simulink model "gm_sampleModel1517_2_sub"  (R2023a)
settings: Solver=VariableStepAuto  StartTime=0.0  StopTime=10.0  RelTol=1e-3
libraries: simulink x1
settings Model: Creator=user1  LastModifiedBy=user1
settings OptimizationCC: BlockReduction=off  ConditionallyExecuteInputs=off
settings DebuggingCC: InheritedTsInSrcMsg=none

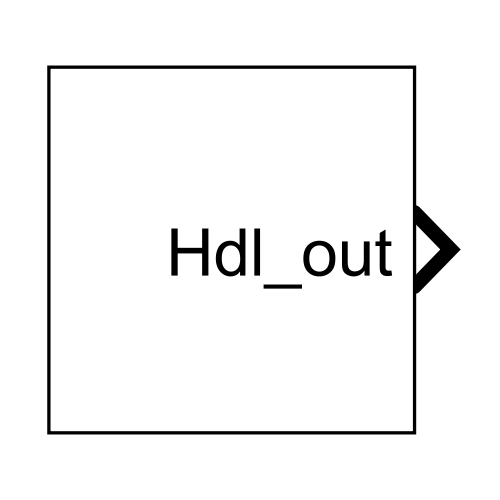
[thumbnail: Simulink's stored preview of the top-level diagram]
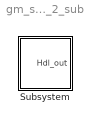
== system gm_sampleModel1517_2_sub ==
  Subsystem : Subsystem

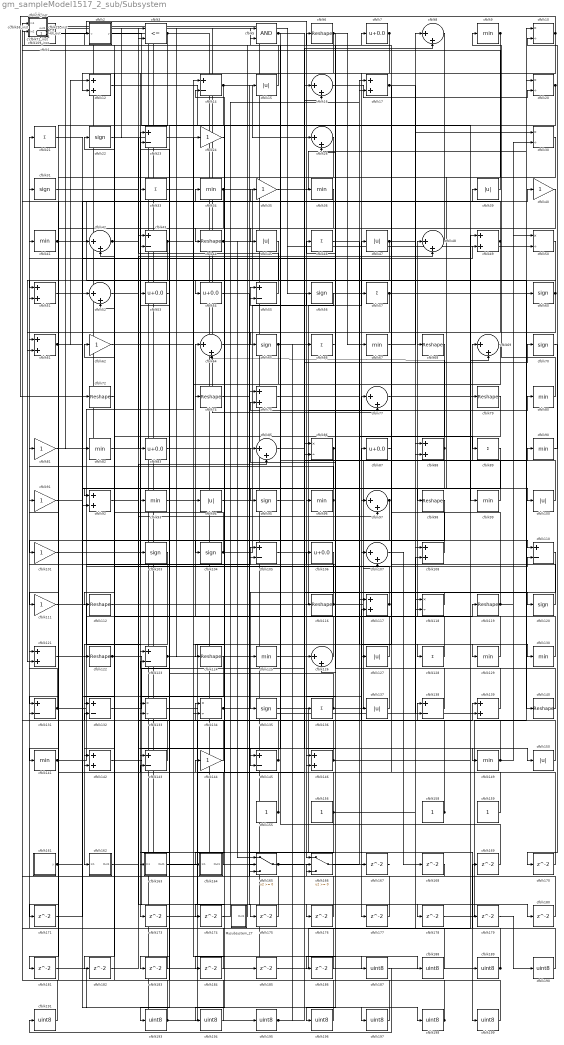
== system gm_sampleModel1517_2_sub/Subsystem ==
  Mysubsystem_27 : Subsystem
  cfblk1 : simulink/Logic and Bit Operations/Extract Bits  bitsToExtract=Upper half  numBits=8  bitIdxRange=[0 7]  outScalingMode=Preserve fixed-point scaling
      settings: LibrarySourceBlock=|
      | hdlsllib/Logic and Bit
      | Operations/Extract Bits
  cfblk{10,20,30,50,86,118,133..134} (8 alike) : Product  Inputs=*/  OutDataTypeStr=uint8  RndMeth=Zero  SaturateOnIntegerOverflow=on
  cfblk{15,39,45,47,94,100,127,137,150} (9 alike) : Abs  OutDataTypeStr=uint8  SaturateOnIntegerOverflow=off
  cfblk{24,35,40,62,81,91,101,111,144} (9 alike) : Gain  OutDataTypeStr=uint8
  cfblk102_inst : Subsystem
  cfblk{22,31,56,60,65,70,95,103..104,120,135} (11 alike) : Signum
  cfblk{14,23,43,55,105,110,123,131..132,138,143,145} (12 alike) : Sum  Inputs=+-  OutDataTypeStr=uint8
  cfblk{7,53..54,83,87,106} (6 alike) : Bias  Bias=0.0  SaturateOnIntegerOverflow=off
  cfblk{8,16,26,42,48,52,64,69,77,85,97,107,126} (13 alike) : Sum  Inputs=|++  OutDataTypeStr=uint8
  cfblk{12,17,49,51,61,75,88,92,108,117,121,139,142,146} (14 alike) : Sum  OutDataTypeStr=uint8
  cfblk109_inst : Subsystem
  cfblk{6,44,68,72,74,79,98,112,116,119,122,124,140} (13 alike) : Reshape
  cfblk{9,34,36,41,67,80,82,90,93,96,99,125,129..130,141,149} (16 alike) : MinMax  OutDataTypeStr=uint8
  cfblk{21,33,46,57,66,89,128,136} (8 alike) : Sum  Inputs=+  OutDataTypeStr=uint8
  cfblk147_inst : Subsystem
  cfblk{155..156,158..159} (4 alike) : Constant  OutDataTypeStr=uint8  SampleTime=-1
  cfblk161 : Subsystem  mask(Counter Free-Running){NumBits=double(16), tsamp=double(-1)}
      mask prompts: NumBits "Simulink:masks:NumberOfBits_MP"; tsamp "Simulink:masks:SampleTime_MP"
      mask help: Simulink:masks:CounterFreeRunning_MD
  cfblk162 : Subsystem
  cfblk163 : Subsystem
  cfblk164 : Subsystem
  cfblk165 : Switch  OutDataTypeStr=uint8  SaturateOnIntegerOverflow=off  InputSameDT=off
  cfblk166 : Switch  OutDataTypeStr=uint8  SaturateOnIntegerOverflow=off  InputSameDT=off
  cfblk{167..171,173..186} (19 alike) : Delay  SampleTime=1
  cfblk{187..191,193..199} (12 alike) : DataTypeConversion  OutDataTypeStr=uint8  SaturateOnIntegerOverflow=off  RndMeth=Floor
  cfblk19_inst : Subsystem
  cfblk2 : Subsystem  mask(Compare To Zero){relop=<=, OutDataTypeStr=uint8, ZeroCross=on}
      mask prompts: relop "Simulink:masks:Operator_MP"; OutDataTypeStr "Simulink:masks:OutputDataType_MP"; ZeroCross "Simulink:masks:EnableZerocrossingDetection_MP"
      mask help: Simulink:masks:CompareToZero_MD
      mask init:
      | OutDataTypeStr = 'uint8';
      | ZeroCross = 'on';
      | blkName = 'sampleModel1517_2_sub/Subsystem/cfblk2';
      | relop = '<=';
      | setValue = 'fixdt(0, 8)';
      mask TypeOptions relop: == | ~= | < | <= | >= | >
      mask TypeOptions OutDataTypeStr: Simulink:masks:uint8 | Simulink:masks:boolean
      mask Callback ZeroCross: sl('zeroCrossEnable', gcbh);
      mask Display: disp([relop,' 0'])
  cfblk29_inst : Subsystem
  cfblk3 : RelationalOperator  Operator=<=  OutDataTypeStr=boolean  InputSameDT=off
  cfblk4 : Constant  Value=0  OutDataTypeStr=uint8  SampleTime=1
  cfblk5 : Logic  AllPortsSameDT=off  OutDataTypeStr=boolean
  cfblk58_inst : Subsystem
  cfblk71_inst : Subsystem
  Hdl_out : Outport  OutDataTypeStr=uint8  SampleTime=1
  wires:
  Mysubsystem_27/1(Out1) -> cfblk71_inst/2(in2)
  cfblk1/1 -> cfblk166/1
  cfblk10/1 -> cfblk72/1, cfblk177/1, cfblk173/1
  cfblk100/1 -> cfblk69/1
  cfblk101/1 -> cfblk23/1
  cfblk102_inst/1(out1) -> cfblk24/1, cfblk185/1
  cfblk103/1 -> cfblk162/1(In1)
  cfblk104/1 -> cfblk56/1, cfblk22/1
  cfblk105/1 -> cfblk80/1
  cfblk106/1 -> cfblk135/1
  cfblk107/1 -> cfblk168/1
  cfblk108/1 -> cfblk87/1
  cfblk109_inst/1(out1) -> cfblk126/1
  cfblk110/1 -> cfblk126/2
  cfblk111/1 -> cfblk123/1
  cfblk112/1 -> cfblk47/1
  cfblk116/1 -> cfblk48/1, cfblk21/1
  cfblk117/1 -> cfblk64/1, cfblk42/2
  cfblk118/1 -> cfblk116/1
  cfblk119/1 -> cfblk75/2, cfblk109_inst/2(in2), cfblk50/1
  cfblk12/1 -> cfblk79/1
  cfblk120/1 -> cfblk33/1
  cfblk121/1 -> cfblk119/1
  cfblk122/1 -> cfblk97/2, cfblk176/1
  cfblk123/1 -> cfblk178/1, cfblk128/1
  cfblk124/1 -> cfblk183/1
  cfblk125/1 -> cfblk8/2
  cfblk126/1 -> cfblk23/2
  cfblk127/1 -> cfblk106/1
  cfblk128/1 -> cfblk68/1
  cfblk129/1 -> cfblk74/1
  cfblk130/1 -> cfblk2/1(u)
  cfblk131/1 -> cfblk51/2, cfblk110/2
  cfblk132/1 -> cfblk90/1
  cfblk133/1 -> cfblk175/1
  cfblk134/1 -> cfblk165/2, cfblk34/1
  cfblk135/1 -> cfblk199/1
  cfblk136/1 -> cfblk107/2, cfblk103/1
  cfblk137/1 -> cfblk105/1
  cfblk138/1 -> cfblk41/1
  cfblk139/1 -> cfblk85/1
  cfblk14/1 -> cfblk26/1, cfblk163/1(In1)
  cfblk140/1 -> cfblk6/1
  cfblk141/1 -> cfblk14/1, cfblk105/2
  cfblk142/1 -> cfblk167/1
  cfblk143/1 -> cfblk147_inst/1(in1)
  cfblk144/1 -> cfblk58_inst/2(in2)
  cfblk145/1 -> cfblk143/1, cfblk134/1
  cfblk146/1 -> cfblk49/1, cfblk62/1
  cfblk147_inst/1(out1) -> cfblk83/1
  cfblk149/1 -> cfblk117/2, cfblk30/2
  cfblk15/1 -> cfblk5/1
  cfblk150/1 -> cfblk138/1
  cfblk155/1 -> cfblk31/1, cfblk143/2
  cfblk156/1 -> cfblk55/1, cfblk165/3, cfblk108/2
  cfblk158/1 -> cfblk61/1, cfblk117/1
  cfblk159/1 -> cfblk77/1
  cfblk16/1 -> cfblk20/2
  cfblk161/1(y) -> cfblk49/2, cfblk40/1
  cfblk162/1(Out1) -> cfblk139/1
  cfblk163/1(Out1) -> cfblk15/1
  cfblk164/1(Out1) -> cfblk144/1
  cfblk165/1 -> cfblk16/1, Hdl_out/1
  cfblk166/1 -> cfblk17/2
  cfblk167/1 -> cfblk1/1
  cfblk168/1 -> cfblk166/2
  cfblk169/1 -> cfblk5/2
  cfblk17/1 -> cfblk118/2, cfblk57/1
  cfblk170/1 -> cfblk14/2
  cfblk171/1 -> cfblk52/1
  cfblk173/1 -> cfblk16/2
  cfblk174/1 -> cfblk17/1
  cfblk175/1 -> cfblk75/1
  cfblk176/1 -> cfblk123/2
  cfblk177/1 -> cfblk166/3
  cfblk178/1 -> cfblk20/1
  cfblk179/1 -> cfblk190/1
  cfblk180/1 -> cfblk58_inst/1(in1)
  cfblk181/1 -> cfblk197/1
  cfblk182/1 -> cfblk85/2
  cfblk183/1 -> cfblk121/1
  cfblk184/1 -> cfblk131/2
  cfblk185/1 -> cfblk69/2
  cfblk186/1 -> cfblk43/2
  cfblk187/1 -> cfblk191/1
  cfblk188/1 -> cfblk93/1
  cfblk189/1 -> cfblk169/1, cfblk118/1
  cfblk19_inst/1(out1) -> cfblk195/1
  cfblk190/1 -> cfblk29_inst/1(in1)
  cfblk191/1 -> cfblk29_inst/2(in2)
  cfblk193/1 -> cfblk71_inst/1(in1), cfblk86/2
  cfblk194/1 -> cfblk53/1
  cfblk195/1 -> cfblk86/1, cfblk66/1
  cfblk196/1 -> cfblk19_inst/1(in1)
  cfblk197/1 -> cfblk19_inst/2(in2)
  cfblk198/1 -> cfblk132/2, cfblk109_inst/1(in1)
  cfblk199/1 -> cfblk91/1
  cfblk2/1(y) -> cfblk88/1
  cfblk20/1 -> cfblk196/1, cfblk184/1
  cfblk21/1 -> cfblk110/1
  cfblk22/1 -> cfblk43/1
  cfblk23/1 -> cfblk94/1
  cfblk24/1 -> cfblk44/1
  cfblk26/1 -> cfblk101/1
  cfblk29_inst/1(out1) -> cfblk189/1
  cfblk3/1 -> cfblk92/1, cfblk181/1
  cfblk30/1 -> cfblk98/1
  cfblk31/1 -> cfblk146/2
  cfblk33/1 -> cfblk188/1
  cfblk34/1 -> cfblk108/1, cfblk171/1
  cfblk35/1 -> cfblk10/1
  cfblk36/1 -> cfblk194/1
  cfblk39/1 -> cfblk102_inst/2(in2)
  cfblk4/1 -> cfblk139/2
  cfblk40/1 -> cfblk127/1
  cfblk41/1 -> cfblk140/1, cfblk35/1
  cfblk42/1 -> cfblk3/2, cfblk182/1
  cfblk43/1 -> cfblk112/1, cfblk130/1
  cfblk44/1 -> cfblk88/2, cfblk165/1
  cfblk45/1 -> cfblk61/2
  cfblk46/1 -> cfblk129/1
  cfblk47/1 -> cfblk138/2, cfblk131/1
  cfblk48/1 -> cfblk45/1
  cfblk49/1 -> cfblk102_inst/1(in1), cfblk133/2
  cfblk5/1 -> cfblk145/2, cfblk120/1
  cfblk50/1 -> cfblk107/1
  cfblk51/1 -> cfblk96/1
  cfblk52/1 -> cfblk54/1
  cfblk53/1 -> cfblk193/1
  cfblk54/1 -> cfblk145/1
  cfblk55/1 -> cfblk3/1
  cfblk56/1 -> cfblk55/2
  cfblk57/1 -> cfblk8/1, cfblk121/2
  cfblk58_inst/1(out1) -> cfblk60/1, cfblk82/1
  cfblk6/1 -> cfblk142/2, cfblk186/1, cfblk67/1
  cfblk60/1 -> cfblk65/1, cfblk51/1, cfblk136/1
  cfblk61/1 -> cfblk137/1, cfblk12/1
  cfblk62/1 -> cfblk97/1
  cfblk64/1 -> cfblk179/1
  cfblk65/1 -> cfblk150/1, cfblk134/2
  cfblk66/1 -> cfblk46/1
  cfblk67/1 -> cfblk30/1
  cfblk68/1 -> cfblk132/1
  cfblk69/1 -> cfblk104/1
  cfblk7/1 -> cfblk12/2, cfblk36/1
  cfblk70/1 -> cfblk170/1
  cfblk71_inst/1(out1) -> cfblk77/2, cfblk50/2
  cfblk72/1 -> cfblk122/1
  cfblk74/1 -> cfblk149/1
  cfblk75/1 -> cfblk89/1
  cfblk77/1 -> cfblk99/1
  cfblk79/1 -> cfblk146/1
  cfblk8/1 -> cfblk142/1
  cfblk80/1 -> cfblk9/1
  cfblk81/1 -> cfblk42/1
  cfblk82/1 -> cfblk48/2
  cfblk83/1 -> cfblk39/1
  cfblk85/1 -> cfblk100/1
  cfblk86/1 -> cfblk26/2, cfblk124/1
  cfblk87/1 -> cfblk7/1
  cfblk88/1 -> cfblk92/2, cfblk64/2
  cfblk89/1 -> cfblk164/1(In1)
  cfblk9/1 -> cfblk95/1, cfblk52/2
  cfblk90/1 -> cfblk10/2
  cfblk91/1 -> cfblk198/1
  cfblk92/1 -> cfblk180/1
  cfblk93/1 -> cfblk187/1
  cfblk94/1 -> cfblk125/1
  cfblk95/1 -> cfblk70/1
  cfblk96/1 -> cfblk81/1, cfblk141/1
  cfblk97/1 -> cfblk174/1, cfblk133/1
  cfblk98/1 -> cfblk111/1
  cfblk99/1 -> cfblk147_inst/2(in2)

== system gm_sampleModel1517_2_sub/Subsystem/Mysubsystem_27 ==
  cfblk157 : Subsystem  mask(Counter Free-Running){NumBits=double(16), tsamp=double(-1)}
      mask prompts: NumBits "Simulink:masks:NumberOfBits_MP"; tsamp "Simulink:masks:SampleTime_MP"
      mask help: Simulink:masks:CounterFreeRunning_MD
  cfblk192 : DataTypeConversion  OutDataTypeStr=uint8  SaturateOnIntegerOverflow=off  RndMeth=Floor
  Out1 : Outport  SampleTime=1
  wires:
  cfblk157/1(y) -> cfblk192/1
  cfblk192/1 -> Out1/1

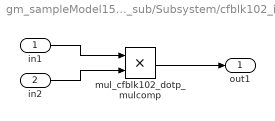
== system gm_sampleModel1517_2_sub/Subsystem/cfblk102_inst ==
  in1 : Inport  OutDataTypeStr=uint8  SampleTime=1
  in2 : Inport  Port=2  OutDataTypeStr=uint8  SampleTime=1
  mul_cfblk102_dotp_mulcomp : Product  Inputs=**  OutDataTypeStr=uint8  SampleTime=1
  out1 : Outport  OutDataTypeStr=uint8  SampleTime=1
  wires:
  in1/1 -> mul_cfblk102_dotp_mulcomp/1
  in2/1 -> mul_cfblk102_dotp_mulcomp/2
  mul_cfblk102_dotp_mulcomp/1 -> out1/1

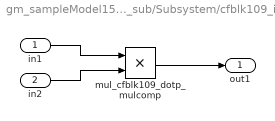
== system gm_sampleModel1517_2_sub/Subsystem/cfblk109_inst ==
  in1 : Inport  OutDataTypeStr=uint8  SampleTime=1
  in2 : Inport  Port=2  OutDataTypeStr=uint8  SampleTime=1
  mul_cfblk109_dotp_mulcomp : Product  Inputs=**  OutDataTypeStr=uint8  SampleTime=1
  out1 : Outport  OutDataTypeStr=uint8  SampleTime=1
  wires:
  in1/1 -> mul_cfblk109_dotp_mulcomp/1
  in2/1 -> mul_cfblk109_dotp_mulcomp/2
  mul_cfblk109_dotp_mulcomp/1 -> out1/1

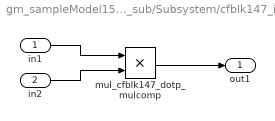
== system gm_sampleModel1517_2_sub/Subsystem/cfblk147_inst ==
  in1 : Inport  OutDataTypeStr=uint8  SampleTime=1
  in2 : Inport  Port=2  OutDataTypeStr=uint8  SampleTime=1
  mul_cfblk147_dotp_mulcomp : Product  Inputs=**  OutDataTypeStr=uint8  SampleTime=1
  out1 : Outport  OutDataTypeStr=uint8  SampleTime=1
  wires:
  in1/1 -> mul_cfblk147_dotp_mulcomp/1
  in2/1 -> mul_cfblk147_dotp_mulcomp/2
  mul_cfblk147_dotp_mulcomp/1 -> out1/1

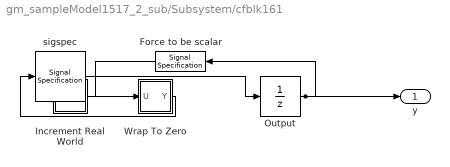
== system gm_sampleModel1517_2_sub/Subsystem/cfblk161 ==
  Force to be scalar : SignalSpecification  DisableCoverage=on  Dimensions=1
  Increment Real World : Subsystem  mask(Real World Value Increment){}
      mask help: Simulink:masks:RealWorldValueIncrement_MD
      mask Display: disp('V++')
  Output : UnitDelay  InitialCondition=0.0  SampleTime=tsamp  HasFrameUpgradeWarning=on
  Wrap To Zero : Subsystem  mask(Wrap To Zero){Threshold=double(65535)}
      mask prompts: Threshold "Simulink:masks:Threshold_MP"
      mask help: Simulink:masks:WrapToZero_MD
  sigspec : SignalSpecification  OutDataTypeStr=uint16  Dimensions=1
  y : Outport  SampleTime=1
  wires:
  Force to be scalar/1 -> Increment Real World/1(u)
  Increment Real World/1(y) -> Wrap To Zero/1(U)
  Output/1 -> Force to be scalar/1, y/1
  Wrap To Zero/1(Y) -> sigspec/1
  sigspec/1 -> Output/1

== system gm_sampleModel1517_2_sub/Subsystem/cfblk162 ==
  In1 : Inport  OutDataTypeStr=uint8  PortDimensions=1  SampleTime=1
  Out1 : Outport  SampleTime=1
  wires:
  In1/1 -> Out1/1

== system gm_sampleModel1517_2_sub/Subsystem/cfblk163 ==
  In1 : Inport  OutDataTypeStr=uint8  PortDimensions=1  SampleTime=1
  Out1 : Outport  SampleTime=1
  wires:
  In1/1 -> Out1/1

== system gm_sampleModel1517_2_sub/Subsystem/cfblk164 ==
  In1 : Inport  OutDataTypeStr=uint8  PortDimensions=1  SampleTime=1
  Out1 : Outport  SampleTime=1
  wires:
  In1/1 -> Out1/1

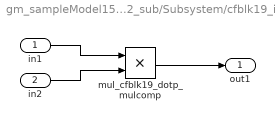
== system gm_sampleModel1517_2_sub/Subsystem/cfblk19_inst ==
  in1 : Inport  OutDataTypeStr=uint8  SampleTime=1
  in2 : Inport  Port=2  OutDataTypeStr=uint8  SampleTime=1
  mul_cfblk19_dotp_mulcomp : Product  Inputs=**  OutDataTypeStr=uint8  SampleTime=1
  out1 : Outport  OutDataTypeStr=uint8  SampleTime=1
  wires:
  in1/1 -> mul_cfblk19_dotp_mulcomp/1
  in2/1 -> mul_cfblk19_dotp_mulcomp/2
  mul_cfblk19_dotp_mulcomp/1 -> out1/1

== system gm_sampleModel1517_2_sub/Subsystem/cfblk2 ==
  u : Inport  OutDataTypeStr=uint8  SampleTime=1
  Compare : RelationalOperator  Operator=<=  OutDataTypeStr=fixdt(0, 8)
  Constant : Constant  DisableCoverage=on  Value=0  OutDataTypeStr=Inherit: Inherit via back propagation  SampleTime=-1  PreserveConstantTs=on
  y : Outport  SampleTime=1
  wires:
  u/1 -> Compare/1
  Compare/1 -> y/1
  Constant/1 -> Compare/2

== system gm_sampleModel1517_2_sub/Subsystem/cfblk29_inst ==
  in1 : Inport  OutDataTypeStr=uint8  SampleTime=1
  in2 : Inport  Port=2  OutDataTypeStr=uint8  SampleTime=1
  mul_cfblk29_dotp_mulcomp : Product  Inputs=**  OutDataTypeStr=uint8  SampleTime=1
  out1 : Outport  OutDataTypeStr=uint8  SampleTime=1
  wires:
  in1/1 -> mul_cfblk29_dotp_mulcomp/1
  in2/1 -> mul_cfblk29_dotp_mulcomp/2
  mul_cfblk29_dotp_mulcomp/1 -> out1/1

== system gm_sampleModel1517_2_sub/Subsystem/cfblk58_inst ==
  in1 : Inport  OutDataTypeStr=uint8  SampleTime=1
  in2 : Inport  Port=2  OutDataTypeStr=uint8  SampleTime=1
  mul_cfblk58_dotp_mulcomp : Product  Inputs=**  OutDataTypeStr=uint8  SampleTime=1
  out1 : Outport  OutDataTypeStr=uint8  SampleTime=1
  wires:
  in1/1 -> mul_cfblk58_dotp_mulcomp/1
  in2/1 -> mul_cfblk58_dotp_mulcomp/2
  mul_cfblk58_dotp_mulcomp/1 -> out1/1

== system gm_sampleModel1517_2_sub/Subsystem/cfblk71_inst ==
  in1 : Inport  OutDataTypeStr=uint8  SampleTime=1
  in2 : Inport  Port=2  OutDataTypeStr=uint8  SampleTime=1
  mul_cfblk71_dotp_mulcomp : Product  Inputs=**  OutDataTypeStr=uint8  SampleTime=1
  out1 : Outport  OutDataTypeStr=uint8  SampleTime=1
  wires:
  in1/1 -> mul_cfblk71_dotp_mulcomp/1
  in2/1 -> mul_cfblk71_dotp_mulcomp/2
  mul_cfblk71_dotp_mulcomp/1 -> out1/1

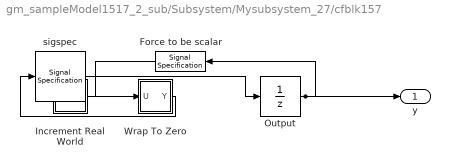
== system gm_sampleModel1517_2_sub/Subsystem/Mysubsystem_27/cfblk157 ==
  Force to be scalar : SignalSpecification  DisableCoverage=on  Dimensions=1
  Increment Real World : Subsystem  mask(Real World Value Increment){}
      mask help: Simulink:masks:RealWorldValueIncrement_MD
      mask Display: disp('V++')
  Output : UnitDelay  InitialCondition=0.0  SampleTime=tsamp  HasFrameUpgradeWarning=on
  Wrap To Zero : Subsystem  mask(Wrap To Zero){Threshold=double(65535)}
      mask prompts: Threshold "Simulink:masks:Threshold_MP"
      mask help: Simulink:masks:WrapToZero_MD
  sigspec : SignalSpecification  OutDataTypeStr=uint16  Dimensions=1
  y : Outport  SampleTime=1
  wires:
  Force to be scalar/1 -> Increment Real World/1(u)
  Increment Real World/1(y) -> Wrap To Zero/1(U)
  Output/1 -> Force to be scalar/1, y/1
  Wrap To Zero/1(Y) -> sigspec/1
  sigspec/1 -> Output/1

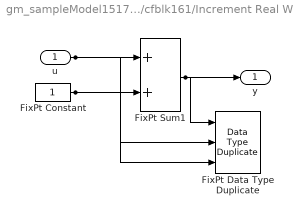
== system gm_sampleModel1517_2_sub/Subsystem/cfblk161/Increment Real World ==
  u : Inport  OutDataTypeStr=uint16  SampleTime=1
  FixPt Constant : Constant  DisableCoverage=on  OutDataTypeStr=Inherit: Inherit via back propagation  SampleTime=-1
  FixPt Data Type Duplicate : DataTypeDuplicate  DisableCoverage=on  NumInputPorts=3
  FixPt Sum1 : Sum  InputSameDT=on  OutDataTypeStr=Inherit: Inherit via back propagation  LockScale=on
  y : Outport  SampleTime=1
  wires:
  u/1 -> FixPt Sum1/1, FixPt Data Type Duplicate/2
  FixPt Constant/1 -> FixPt Sum1/2, FixPt Data Type Duplicate/3
  FixPt Sum1/1 -> FixPt Data Type Duplicate/1, y/1

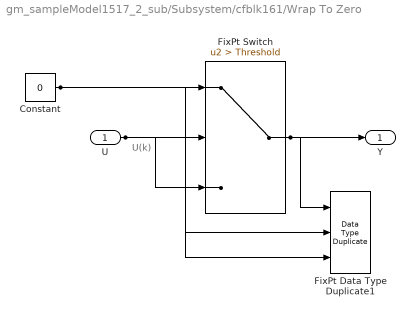
== system gm_sampleModel1517_2_sub/Subsystem/cfblk161/Wrap To Zero ==
  note: U(k)
  U : Inport  OutDataTypeStr=uint16  SampleTime=1
  Constant : Constant  DisableCoverage=on  Value=0  OutDataTypeStr=Inherit: Inherit via back propagation  SampleTime=-1
  FixPt Data Type Duplicate1 : DataTypeDuplicate  DisableCoverage=on  NumInputPorts=3
  FixPt Switch : Switch  Criteria=u2 > Threshold  Threshold=Threshold  OutDataTypeStr=Inherit: Inherit via back propagation  ZeroCross=off  SaturateOnIntegerOverflow=off  InputSameDT=off
  Y : Outport  SampleTime=1
  wires:
  U/1 -> FixPt Switch/3, FixPt Switch/2, FixPt Data Type Duplicate1/2
  Constant/1 -> FixPt Switch/1, FixPt Data Type Duplicate1/3
  FixPt Switch/1 -> FixPt Data Type Duplicate1/1, Y/1

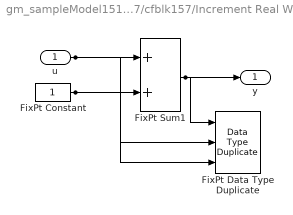
== system gm_sampleModel1517_2_sub/Subsystem/Mysubsystem_27/cfblk157/Increment Real World ==
  u : Inport  OutDataTypeStr=uint16  SampleTime=1
  FixPt Constant : Constant  DisableCoverage=on  OutDataTypeStr=Inherit: Inherit via back propagation  SampleTime=-1
  FixPt Data Type Duplicate : DataTypeDuplicate  DisableCoverage=on  NumInputPorts=3
  FixPt Sum1 : Sum  InputSameDT=on  OutDataTypeStr=Inherit: Inherit via back propagation  LockScale=on
  y : Outport  SampleTime=1
  wires:
  u/1 -> FixPt Sum1/1, FixPt Data Type Duplicate/2
  FixPt Constant/1 -> FixPt Sum1/2, FixPt Data Type Duplicate/3
  FixPt Sum1/1 -> FixPt Data Type Duplicate/1, y/1

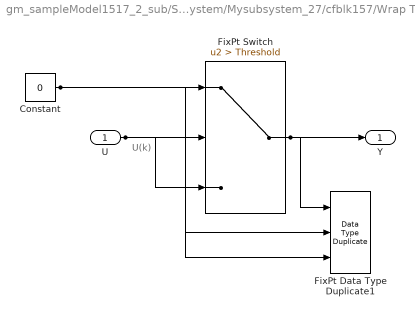
== system gm_sampleModel1517_2_sub/Subsystem/Mysubsystem_27/cfblk157/Wrap To Zero ==
  note: U(k)
  U : Inport  OutDataTypeStr=uint16  SampleTime=1
  Constant : Constant  DisableCoverage=on  Value=0  OutDataTypeStr=Inherit: Inherit via back propagation  SampleTime=-1
  FixPt Data Type Duplicate1 : DataTypeDuplicate  DisableCoverage=on  NumInputPorts=3
  FixPt Switch : Switch  Criteria=u2 > Threshold  Threshold=Threshold  OutDataTypeStr=Inherit: Inherit via back propagation  ZeroCross=off  SaturateOnIntegerOverflow=off  InputSameDT=off
  Y : Outport  SampleTime=1
  wires:
  U/1 -> FixPt Switch/3, FixPt Switch/2, FixPt Data Type Duplicate1/2
  Constant/1 -> FixPt Switch/1, FixPt Data Type Duplicate1/3
  FixPt Switch/1 -> FixPt Data Type Duplicate1/1, Y/1
